simulink model "CruiseControl"  (R2017b)
settings: Solver=VariableStepAuto  StartTime=0.0  StopTime=10.0  RelTol=1e-3
settings Model: Creator=rafae  LastModifiedBy=rafae

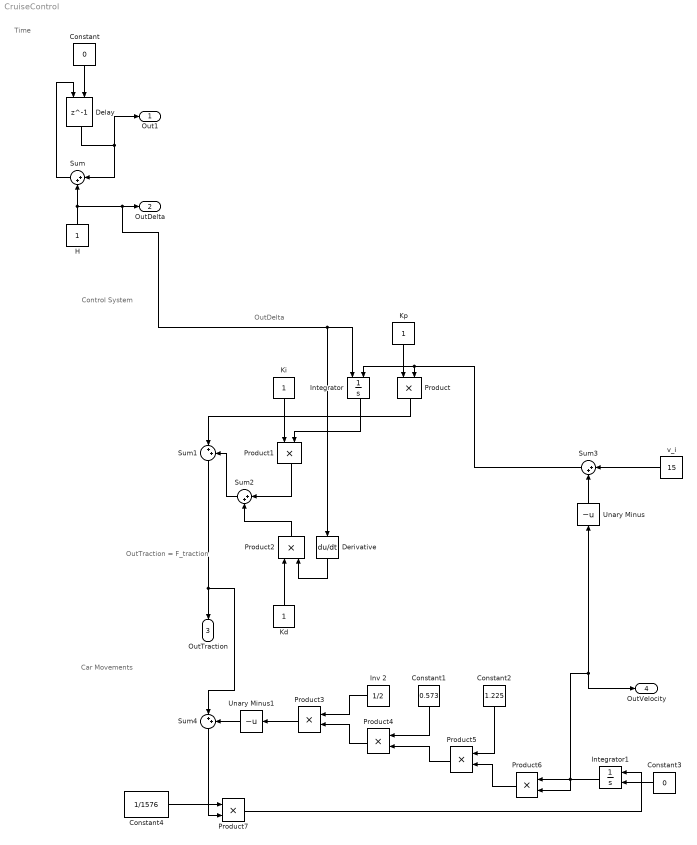
== system CruiseControl ==
  note: Car Movements
  note: Control System
  note: OutDelta
  note: OutTraction = F_traction
  note: Time
  Constant : Constant  Value=0
  Constant1 : Constant  Value=0.573
  Constant2 : Constant  Value=1.225
  Constant3 : Constant  Value=0
  Constant4 : Constant  Value=1/1576
  Delay : Delay  DelayLength=1  InitialConditionSource=Input port  InitialCondition=0
      settings: InputPortMap=u0,p4
  Derivative : Derivative
  "H " : Constant
  Integrator : Integrator  InitialConditionSource=external
  Integrator1 : Integrator  InitialConditionSource=external
  Inv 2 : Constant  Value=1/2
  Kd : Constant
  Ki : Constant
  Kp : Constant
  Product{,1..7} (8 alike) : Product
  Sum{,1..4} (5 alike) : Sum  Inputs=|++
  Unary Minus : UnaryMinus
  Unary Minus1 : UnaryMinus
  v_i : Constant  Value=15
  Out1 : Outport
  "OutDelta " : Outport  Port=2
  OutTraction : Outport  Port=3
  OutVelocity : Outport  Port=4
  wires:
  Delay/1 -> Sum/1, Out1/1
  Constant/1 -> Delay/2
  Sum/1 -> Delay/1
  "H "/1 -> Sum/2, Derivative/1, Integrator/1, "OutDelta "/1
  Kp/1 -> Product/1
  Ki/1 -> Product1/1
  Product/1 -> Sum1/1
  Sum1/1 -> Sum4/1, OutTraction/1
  Sum2/1 -> Sum1/2
  Product1/1 -> Sum2/1
  Product2/1 -> Sum2/2
  Kd/1 -> Product2/1
  Integrator/1 -> Product1/2
  Derivative/1 -> Product2/2
  Sum3/1 -> Integrator/2, Product/2
  v_i/1 -> Sum3/1
  Unary Minus/1 -> Sum3/2
  Integrator1/1 -> Unary Minus/1, OutVelocity/1, Product6/2, Product6/1
  Unary Minus1/1 -> Sum4/2
  Product3/1 -> Unary Minus1/1
  Inv 2/1 -> Product3/1
  Product4/1 -> Product3/2
  Constant1/1 -> Product4/1
  Product5/1 -> Product4/2
  Constant2/1 -> Product5/1
  Product6/1 -> Product5/2
  Constant3/1 -> Integrator1/2
  Product7/1 -> Integrator1/1
  Sum4/1 -> Product7/2
  Constant4/1 -> Product7/1
